simulink model "DC_Motor_Control_System"  (R2024b)
settings: Solver=VariableStepAuto  StartTime=0.0  StopTime=10  RelTol=1e-3
undefined symbols (not defined in the file or in its folder): controllerGain, motorGain, motorTimeConstant
settings Model: Creator=elias  LastModifiedBy=elias

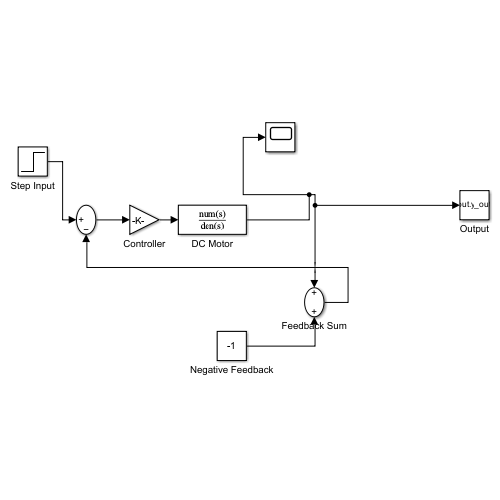
[thumbnail: Simulink's stored preview of the top-level diagram]
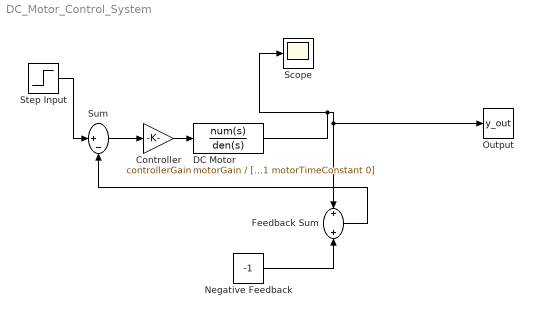
== system DC_Motor_Control_System ==
  Controller : Gain  Gain=controllerGain
  DC Motor : TransferFcn  Numerator=motorGain  Denominator=[1 motorTimeConstant 0]
  Feedback Sum : Sum
  Negative Feedback : Constant  Value=-1
  Output : ToWorkspace  VariableName=y_out  SaveFormat=Timeseries  SampleTime=-1
  Scope : Scope
  Step Input : Step  SampleTime=0
  Sum : Sum  Inputs=|+-
  wires:
  Step Input/1 -> Sum/1
  Sum/1 -> Controller/1
  Controller/1 -> DC Motor/1
  DC Motor/1 -> Feedback Sum/1, Output/1, Scope/1
  Feedback Sum/1 -> Sum/2
  Negative Feedback/1 -> Feedback Sum/2
